simulink model "integration_PID_model_3"  (R2023a)
settings: Solver=VariableStepAuto  StartTime=0.0  StopTime=30  FixedStep=1e-3  RelTol=1e-3
PreLoadFcn:
  | %
  | 
  | %   Copyright 2020-2022 The MathWorks, Inc.
  | 
  | %Based on the quadcopter model used in jMAVSim
  | 
  | Ixx = 0.005; %Kgm^2
  | Iyy = 0.005;
  | Izz = 0.009;
  | 
  | 
  | inertia = diag([Ixx, Iyy, Izz]);
  | 
  | mass = 0.8; %Kg
  | g = 9.81; %m/s^2
  | 
  | armLength = 0.33/2; % length of Arm measured from center in m
  | 
  | rotorThrustMax = 4; %N
  | 
  | rotorTorqueMax = 0.05 ;%Nm
  | 
  | rotorTimeConst = 0.005 ;% time constant of rotor (motor + propeller)
  | 
  | %rotorOffset = [0 0 0]; % Rotors position offsets from Gravity center
  | 
  | dragCoeffMov = 0.01; %drag coefficient for linear motion of quadcopter
  | windVel = [0 0 0]';
  | 
  | % Initial states
  | init.posNED = [0, 0, 0]; % m
  | init.vb = [0 0 0]'; %m/s
  | init.euler = [0, 0, 0]'; %Roll Pitch Yaw Rads
  | init.angRates = [0, 0, 0]; %rad/s
  | 
  | 
  | %Computed from above values
  | rotorPositions = zeros(3,4);
  | axisD = armLength/sqrt(2);
  | rotorPositions(:,1) = [axisD, axisD, 0]';
  | rotorPositions(:,2) = [-axisD, -axisD, 0]';
  | rotorPositions(:,3) = [+axisD, -axisD, 0]';
  | rotorPositions(:,4) = [-axisD, axisD, 0]';
  | rotorDir = [-1, -1, 1, 1]; %rotation direction. +ve = clockwise
  | 
  | % Sample Time
  | SampleTime = 0.008;
  | 
  | %Gain to convert m to mm
  | m_to_mm = 1000;
  | 
  | %Gain to convert m/s^2 to mG
  | ms2_to_mg = (1/9.80665)*1000;
  | 
  | %Gain to convert m/s to cm/s
  | ms_to_cms = 100;
  | 
  | %Reference height for 'Flat Earth to LLA'
  | ref_height = -71.3232;
  | 
  | ... (+137 lines)
values from neighbouring files (symbols this model uses):
  delay_tilt = 0.004    [integration_parameters.m]    (also in simulation_parameters.m)
  kf = 65    [integration_parameters.m]    (also in simulation_parameters.m)
  Lh = 0.2    [CoG_shift.m]    (also in integration_parameters.m; simulation_parameters.m)
  Lv = 0.2    [integration_parameters.m]    (also in simulation_parameters.m)
  m = 1.12    [integration_parameters.m]    (also in optimal_controller_pitching.m; simulation_parameters.m)
  N = 150    [MPC_controller_full.m]
  p_D = 0    [controller_parameters.m]    (also in integration_parameters.m)
  p_I = 0    [controller_parameters.m]    (also in integration_parameters.m)
  p_P = 0.35    [controller_parameters.m]    (also in integration_parameters.m)
  pitch_D = 0    [controller_parameters.m]    (also in integration_parameters.m)
  pitch_I = 0.05    [controller_parameters.m]    (also in integration_parameters.m = 0)
  pitch_P = 2    [controller_parameters.m]    (also in integration_parameters.m = 10)
  q_D = 0    [controller_parameters.m]    (also in integration_parameters.m)
  q_I = 0    [controller_parameters.m]    (also in integration_parameters.m)
  q_P = 1.5    [controller_parameters.m]    (also in integration_parameters.m = 10)
  r_D = 0    [controller_parameters.m]    (also in integration_parameters.m)
  r_I = 0    [controller_parameters.m]    (also in integration_parameters.m)
  r_P = 1    [controller_parameters.m]    (also in integration_parameters.m)
  reference = [1 1 1 0 30 60]'    [integration_parameters.m]    (also in simulation_parameters.m = [1 1 1 0 30 40]')
  roll_D = 1    [controller_parameters.m]    (also in integration_parameters.m)
  roll_I = 0    [controller_parameters.m]    (also in integration_parameters.m)
  roll_P = 8    [controller_parameters.m]    (also in integration_parameters.m)
  s_r = [1 1 1 1 1 1]    [integration_parameters.m]    (also in simulation_parameters.m)
  Tmax = 5.5    [integration_parameters.m]    (also in simulation_parameters.m)
  vx_D = 0    [controller_parameters.m]
  vx_I = 0    [controller_parameters.m]
  vx_P = 10    [controller_parameters.m]
  vy_D = 0    [controller_parameters.m]    (also in integration_parameters.m)
  vy_I = 0    [controller_parameters.m]    (also in integration_parameters.m)
  vy_P = 12    [controller_parameters.m]    (also in integration_parameters.m)
  vz_D = 0    [controller_parameters.m]    (also in integration_parameters.m)
  vz_I = 0    [controller_parameters.m]    (also in integration_parameters.m)
  vz_P = 8    [controller_parameters.m]    (also in integration_parameters.m = 9)
  x_D = 1.5    [controller_parameters.m]    (also in integration_parameters.m = 0)
  x_I = 0    [controller_parameters.m]    (also in integration_parameters.m)
  x_P = 6    [controller_parameters.m]    (also in integration_parameters.m = 1.5)
  y_D = 0.3    [controller_parameters.m]    (also in integration_parameters.m)
  y_I = 0    [controller_parameters.m]    (also in integration_parameters.m)
  y_P = 1.5    [controller_parameters.m]    (also in integration_parameters.m)
  yaw_D = 0    [controller_parameters.m]    (also in integration_parameters.m)
  yaw_I = 0    [controller_parameters.m]    (also in integration_parameters.m)
  yaw_P = 1.5    [controller_parameters.m]    (also in integration_parameters.m)
  z_D = 0    [controller_parameters.m]    (also in integration_parameters.m)
  z_I = 0    [controller_parameters.m]    (also in integration_parameters.m)
  z_P = 3    [controller_parameters.m]    (also in integration_parameters.m = 2.5)
undefined symbols (not defined in the file or in its folder): X, Y, Z
libraries: sm_lib x47, nesl_utility x23, slpidlib x12, simulink x5, simulink_extras x4, SignalEditorBlockLib x1
(part 2 of 4)

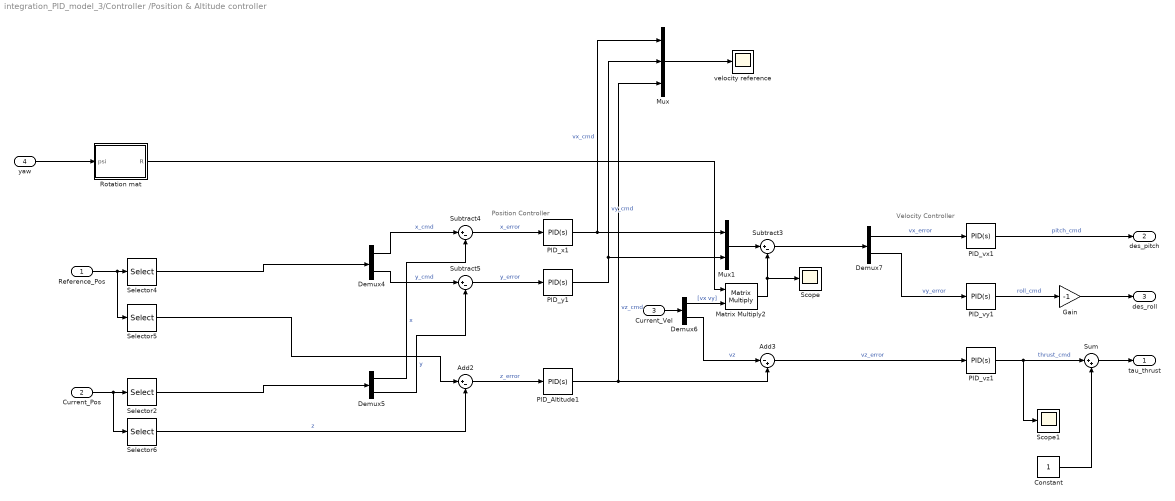
== system integration_PID_model_3/Controller /Position & Altitude controller ==
  note: Position Controller
  note: Velocity Controller
  Reference_Pos : Inport
  Current_Pos : Inport  Port=2
  Current_Vel : Inport  Port=3
  yaw : Inport  Port=4
  Add2 : Sum  Inputs=|+-
  Add3 : Sum  Inputs=|-+
  Constant : Constant
  Demux4 : Demux  Outputs=2
  Demux5 : Demux  Outputs=2
  Demux6 : Demux  Outputs=[2 1]
  Demux7 : Demux  Outputs=2
  Gain : Gain  Gain=-1
  Matrix Multiply2 : Product  Multiplication=Matrix(*)
  Mux : Mux  Inputs=3
  Mux1 : Mux  Inputs=2
  PID_Altitude1 : slpidlib/PID Controller  Controller=PID  Form=Parallel  TimeDomain=Continuous-time  UseExternalTs=off  SampleTime=-1  IntegratorMethod=Backward Euler  FilterMethod=Forward Euler  ControllerParametersSource=internal  P=z_P  I=z_I  UseKiTs=off  D=z_D  N=100  UseFilter=on  TunerSelectOption=Transfer Function Based (PID Tuner App)  InitialConditionSource=internal  InitialConditionForIntegrator=0  InitialConditionForFilter=0  DifferentiatorICPrevScaledInput=0  ExternalReset=none  TrackingMode=off  Kt=1  LimitOutput=on  SatLimitsSource=internal  UpperSaturationLimit=10  LowerSaturationLimit=-10  LinearizeAsGain=off  AntiWindupMode=clamping  Kb=1  LimitIntegrator=off  UpperIntegratorSaturationLimit=inf  LowerIntegratorSaturationLimit=-inf  POutMin=[]  POutMax=[]  IOutMin=[]  IOutMax=[]  DOutMin=[]  DOutMax=[]  NOutMin=[]  NOutMax=[]  SumOutMin=[]  SumOutMax=[]  SaturationOutMin=[]  SaturationOutMax=[]  PParamMin=[]  PParamMax=[]  IParamMin=[]  IParamMax=[]  DParamMin=[]  DParamMax=[]  NParamMin=[]  NParamMax=[]  KbParamMin=[]  KbParamMax=[]  KtParamMin=[]  KtParamMax=[]  KbOutMin=[]  KbOutMax=[]  KtOutMin=[]  KtOutMax=[]  IntegratorOutMin=[]  IntegratorOutMax=[]  FilterOutMin=[]  FilterOutMax=[]  SumI1OutMin=[]  SumI1OutMax=[]  SumI2OutMin=[]  SumI2OutMax=[]  SumI3OutMin=[]  SumI3OutMax=[]  SumI4OutMin=[]  SumI4OutMax=[]  SumDOutMin=[]  SumDOutMax=[]  DifferentiatorOutMin=[]  DifferentiatorOutMax=[]  FilterDiffOutCoefMin=[]  FilterDiffOutCoefMax=[]  ReciprocalOutMin=[]  ReciprocalOutMax=[]  SumDenOutMin=[]  SumDenOutMax=[]  SumNumOutMin=[]  SumNumOutMax=[]  DivideOutMin=[]  DivideOutMax=[]  UdiffTsProdOutMin=[]  UdiffTsProdOutMax=[]  NTsProdOutMin=[]  NTsProdOutMax=[]  UintegralTsProdOutMin=[]  UintegralTsProdOutMax=[]  UngainTsProdOutMin=[]  UngainTsProdOutMax=[]  ClampingZeroOutDataTypeStr=Inherit: Inherit via back propagation  ClampingZeroOutMin=[]  ClampingZeroOutMax=[]  FilterDenConstantOutDataTypeStr=Inherit: Inherit via back propagation  FilterDenConstantOutMin=[]  FilterDenConstantOutMax=[]  PCopyOutDataTypeStr=Inherit: Inherit via back propagation  PCopyOutMin=[]  PCopyOutMax=[]  NCopyOutDataTypeStr=Inherit: Inherit via back propagation  NCopyOutMin=[]  NCopyOutMax=[]  IntegratorContinuousStateAttributes=''  IntegratorStateMustResolveToSignalObject=off  IntegratorRTWStateStorageClass=Auto  FilterContinuousStateAttributes=''  FilterStateMustResolveToSignalObject=off  FilterRTWStateStorageClass=Auto  ParallelPVariant=InternalParameters  IdealPVariant=Disabled  IVariant=InternalParameters  DVariant=InternalParameters  IntegratorVariant=Continuous  SatVariant=Enabled  AWVariant=ContClampingParallel  PCopyVariant=Disabled  TRVariant=Disabled  FdbkBlocksVariant=Forward  IdealPFdbkVariant=Disabled  SatFdbkVariant=Disabled  DerivativeFilterVariant=ContFilter  NVariant=InternalParameters  NCopyVariant=Disabled  FilterICVariant=InternalICsFilter  IntegratorICVariant=InternalICs  ExternalResetVariant=Disabled  TRSumVariant=Passthrough  SumFdbkVariant=Disabled  SumVariant=Sum_PID  TsampFilterVariant=InternalTs  TsampNgainVariant=Passthrough  TsampIntegralVariant=Disabled_SignalSpec  ExternalSaturationOutDataTypeStr=Inherit: Same as second input
  PID_vx1 : slpidlib/PID Controller  Controller=PID  Form=Parallel  TimeDomain=Continuous-time  UseExternalTs=off  SampleTime=-1  IntegratorMethod=Forward Euler  FilterMethod=Forward Euler  ControllerParametersSource=internal  P=vx_P  I=vx_I  UseKiTs=off  D=vx_D  N=100  UseFilter=on  TunerSelectOption=Transfer Function Based (PID Tuner App)  InitialConditionSource=internal  InitialConditionForIntegrator=0  InitialConditionForFilter=0  DifferentiatorICPrevScaledInput=0  ExternalReset=none  TrackingMode=off  Kt=1  LimitOutput=on  SatLimitsSource=internal  UpperSaturationLimit=50  LowerSaturationLimit=-50  LinearizeAsGain=off  AntiWindupMode=none  Kb=1  LimitIntegrator=off  UpperIntegratorSaturationLimit=inf  LowerIntegratorSaturationLimit=-inf  POutMin=[]  POutMax=[]  IOutMin=[]  IOutMax=[]  DOutMin=[]  DOutMax=[]  NOutMin=[]  NOutMax=[]  SumOutMin=[]  SumOutMax=[]  SaturationOutMin=[]  SaturationOutMax=[]  PParamMin=[]  PParamMax=[]  IParamMin=[]  IParamMax=[]  DParamMin=[]  DParamMax=[]  NParamMin=[]  NParamMax=[]  KbParamMin=[]  KbParamMax=[]  KtParamMin=[]  KtParamMax=[]  KbOutMin=[]  KbOutMax=[]  KtOutMin=[]  KtOutMax=[]  IntegratorOutMin=[]  IntegratorOutMax=[]  FilterOutMin=[]  FilterOutMax=[]  SumI1OutMin=[]  SumI1OutMax=[]  SumI2OutMin=[]  SumI2OutMax=[]  SumI3OutMin=[]  SumI3OutMax=[]  SumI4OutMin=[]  SumI4OutMax=[]  SumDOutMin=[]  SumDOutMax=[]  DifferentiatorOutMin=[]  DifferentiatorOutMax=[]  FilterDiffOutCoefMin=[]  FilterDiffOutCoefMax=[]  ReciprocalOutMin=[]  ReciprocalOutMax=[]  SumDenOutMin=[]  SumDenOutMax=[]  SumNumOutMin=[]  SumNumOutMax=[]  DivideOutMin=[]  DivideOutMax=[]  UdiffTsProdOutMin=[]  UdiffTsProdOutMax=[]  NTsProdOutMin=[]  NTsProdOutMax=[]  UintegralTsProdOutMin=[]  UintegralTsProdOutMax=[]  UngainTsProdOutMin=[]  UngainTsProdOutMax=[]  ClampingZeroOutDataTypeStr=Inherit: Inherit via back propagation  ClampingZeroOutMin=[]  ClampingZeroOutMax=[]  FilterDenConstantOutDataTypeStr=Inherit: Inherit via back propagation  FilterDenConstantOutMin=[]  FilterDenConstantOutMax=[]  PCopyOutDataTypeStr=Inherit: Inherit via back propagation  PCopyOutMin=[]  PCopyOutMax=[]  NCopyOutDataTypeStr=Inherit: Inherit via back propagation  NCopyOutMin=[]  NCopyOutMax=[]  IntegratorContinuousStateAttributes=''  IntegratorStateMustResolveToSignalObject=off  IntegratorRTWStateStorageClass=Auto  FilterContinuousStateAttributes=''  FilterStateMustResolveToSignalObject=off  FilterRTWStateStorageClass=Auto  ParallelPVariant=InternalParameters  IdealPVariant=Disabled  IVariant=InternalParameters  DVariant=InternalParameters  IntegratorVariant=Continuous  SatVariant=Enabled  AWVariant=Passthrough  PCopyVariant=Disabled  TRVariant=Disabled  FdbkBlocksVariant=Forward  IdealPFdbkVariant=Disabled  SatFdbkVariant=Disabled  DerivativeFilterVariant=ContFilter  NVariant=InternalParameters  NCopyVariant=Disabled  FilterICVariant=InternalICsFilter  IntegratorICVariant=InternalICs  ExternalResetVariant=Disabled  TRSumVariant=Passthrough  SumFdbkVariant=Disabled  SumVariant=Sum_PID  TsampFilterVariant=InternalTs  TsampNgainVariant=Passthrough  TsampIntegralVariant=Disabled_SignalSpec  ExternalSaturationOutDataTypeStr=Inherit: Same as second input
  PID_vy1 : slpidlib/PID Controller  Controller=PID  Form=Parallel  TimeDomain=Continuous-time  UseExternalTs=off  SampleTime=-1  IntegratorMethod=Forward Euler  FilterMethod=Forward Euler  ControllerParametersSource=internal  P=vy_P  I=vy_I  UseKiTs=off  D=vy_D  N=100  UseFilter=on  TunerSelectOption=Frequency Response Based  InitialConditionSource=internal  InitialConditionForIntegrator=0  InitialConditionForFilter=0  DifferentiatorICPrevScaledInput=0  ExternalReset=none  TrackingMode=off  Kt=1  LimitOutput=on  SatLimitsSource=internal  UpperSaturationLimit=50  LowerSaturationLimit=-50  LinearizeAsGain=off  AntiWindupMode=none  Kb=1  LimitIntegrator=off  UpperIntegratorSaturationLimit=inf  LowerIntegratorSaturationLimit=-inf  POutMin=[]  POutMax=[]  IOutMin=[]  IOutMax=[]  DOutMin=[]  DOutMax=[]  NOutMin=[]  NOutMax=[]  SumOutMin=[]  SumOutMax=[]  SaturationOutMin=[]  SaturationOutMax=[]  PParamMin=[]  PParamMax=[]  IParamMin=[]  IParamMax=[]  DParamMin=[]  DParamMax=[]  NParamMin=[]  NParamMax=[]  KbParamMin=[]  KbParamMax=[]  KtParamMin=[]  KtParamMax=[]  KbOutMin=[]  KbOutMax=[]  KtOutMin=[]  KtOutMax=[]  IntegratorOutMin=[]  IntegratorOutMax=[]  FilterOutMin=[]  FilterOutMax=[]  SumI1OutMin=[]  SumI1OutMax=[]  SumI2OutMin=[]  SumI2OutMax=[]  SumI3OutMin=[]  SumI3OutMax=[]  SumI4OutMin=[]  SumI4OutMax=[]  SumDOutMin=[]  SumDOutMax=[]  DifferentiatorOutMin=[]  DifferentiatorOutMax=[]  FilterDiffOutCoefMin=[]  FilterDiffOutCoefMax=[]  ReciprocalOutMin=[]  ReciprocalOutMax=[]  SumDenOutMin=[]  SumDenOutMax=[]  SumNumOutMin=[]  SumNumOutMax=[]  DivideOutMin=[]  DivideOutMax=[]  UdiffTsProdOutMin=[]  UdiffTsProdOutMax=[]  NTsProdOutMin=[]  NTsProdOutMax=[]  UintegralTsProdOutMin=[]  UintegralTsProdOutMax=[]  UngainTsProdOutMin=[]  UngainTsProdOutMax=[]  ClampingZeroOutDataTypeStr=Inherit: Inherit via back propagation  ClampingZeroOutMin=[]  ClampingZeroOutMax=[]  FilterDenConstantOutDataTypeStr=Inherit: Inherit via back propagation  FilterDenConstantOutMin=[]  FilterDenConstantOutMax=[]  PCopyOutDataTypeStr=Inherit: Inherit via back propagation  PCopyOutMin=[]  PCopyOutMax=[]  NCopyOutDataTypeStr=Inherit: Inherit via back propagation  NCopyOutMin=[]  NCopyOutMax=[]  IntegratorContinuousStateAttributes=''  IntegratorStateMustResolveToSignalObject=off  IntegratorRTWStateStorageClass=Auto  FilterContinuousStateAttributes=''  FilterStateMustResolveToSignalObject=off  FilterRTWStateStorageClass=Auto  ParallelPVariant=InternalParameters  IdealPVariant=Disabled  IVariant=InternalParameters  DVariant=InternalParameters  IntegratorVariant=Continuous  SatVariant=Enabled  AWVariant=Passthrough  PCopyVariant=Disabled  TRVariant=Disabled  FdbkBlocksVariant=Forward  IdealPFdbkVariant=Disabled  SatFdbkVariant=Disabled  DerivativeFilterVariant=ContFilter  NVariant=InternalParameters  NCopyVariant=Disabled  FilterICVariant=InternalICsFilter  IntegratorICVariant=InternalICs  ExternalResetVariant=Disabled  TRSumVariant=Passthrough  SumFdbkVariant=Disabled  SumVariant=Sum_PID  TsampFilterVariant=InternalTs  TsampNgainVariant=Passthrough  TsampIntegralVariant=Disabled_SignalSpec  ExternalSaturationOutDataTypeStr=Inherit: Same as second input
  PID_vz1 : slpidlib/PID Controller  Controller=PID  Form=Parallel  TimeDomain=Continuous-time  UseExternalTs=off  SampleTime=-1  IntegratorMethod=Backward Euler  FilterMethod=Forward Euler  ControllerParametersSource=internal  P=vz_P  I=vz_I  UseKiTs=off  D=vz_D  N=100  UseFilter=on  TunerSelectOption=Transfer Function Based (PID Tuner App)  InitialConditionSource=internal  InitialConditionForIntegrator=0  InitialConditionForFilter=0  DifferentiatorICPrevScaledInput=0  ExternalReset=none  TrackingMode=off  Kt=1  LimitOutput=off  SatLimitsSource=internal  UpperSaturationLimit=2  LowerSaturationLimit=0  LinearizeAsGain=off  AntiWindupMode=none  Kb=1  LimitIntegrator=off  UpperIntegratorSaturationLimit=inf  LowerIntegratorSaturationLimit=-inf  POutMin=[]  POutMax=[]  IOutMin=[]  IOutMax=[]  DOutMin=[]  DOutMax=[]  NOutMin=[]  NOutMax=[]  SumOutMin=[]  SumOutMax=[]  SaturationOutMin=[]  SaturationOutMax=[]  PParamMin=[]  PParamMax=[]  IParamMin=[]  IParamMax=[]  DParamMin=[]  DParamMax=[]  NParamMin=[]  NParamMax=[]  KbParamMin=[]  KbParamMax=[]  KtParamMin=[]  KtParamMax=[]  KbOutMin=[]  KbOutMax=[]  KtOutMin=[]  KtOutMax=[]  IntegratorOutMin=[]  IntegratorOutMax=[]  FilterOutMin=[]  FilterOutMax=[]  SumI1OutMin=[]  SumI1OutMax=[]  SumI2OutMin=[]  SumI2OutMax=[]  SumI3OutMin=[]  SumI3OutMax=[]  SumI4OutMin=[]  SumI4OutMax=[]  SumDOutMin=[]  SumDOutMax=[]  DifferentiatorOutMin=[]  DifferentiatorOutMax=[]  FilterDiffOutCoefMin=[]  FilterDiffOutCoefMax=[]  ReciprocalOutMin=[]  ReciprocalOutMax=[]  SumDenOutMin=[]  SumDenOutMax=[]  SumNumOutMin=[]  SumNumOutMax=[]  DivideOutMin=[]  DivideOutMax=[]  UdiffTsProdOutMin=[]  UdiffTsProdOutMax=[]  NTsProdOutMin=[]  NTsProdOutMax=[]  UintegralTsProdOutMin=[]  UintegralTsProdOutMax=[]  UngainTsProdOutMin=[]  UngainTsProdOutMax=[]  ClampingZeroOutDataTypeStr=Inherit: Inherit via back propagation  ClampingZeroOutMin=[]  ClampingZeroOutMax=[]  FilterDenConstantOutDataTypeStr=Inherit: Inherit via back propagation  FilterDenConstantOutMin=[]  FilterDenConstantOutMax=[]  PCopyOutDataTypeStr=Inherit: Inherit via back propagation  PCopyOutMin=[]  PCopyOutMax=[]  NCopyOutDataTypeStr=Inherit: Inherit via back propagation  NCopyOutMin=[]  NCopyOutMax=[]  IntegratorContinuousStateAttributes=''  IntegratorStateMustResolveToSignalObject=off  IntegratorRTWStateStorageClass=Auto  FilterContinuousStateAttributes=''  FilterStateMustResolveToSignalObject=off  FilterRTWStateStorageClass=Auto  ParallelPVariant=InternalParameters  IdealPVariant=Disabled  IVariant=InternalParameters  DVariant=InternalParameters  IntegratorVariant=Continuous  SatVariant=Disabled  AWVariant=Passthrough  PCopyVariant=Disabled  TRVariant=Disabled  FdbkBlocksVariant=Forward  IdealPFdbkVariant=Disabled  SatFdbkVariant=Disabled  DerivativeFilterVariant=ContFilter  NVariant=InternalParameters  NCopyVariant=Disabled  FilterICVariant=InternalICsFilter  IntegratorICVariant=InternalICs  ExternalResetVariant=Disabled  TRSumVariant=Passthrough  SumFdbkVariant=Disabled  SumVariant=Sum_PID  TsampFilterVariant=InternalTs  TsampNgainVariant=Passthrough  TsampIntegralVariant=Disabled_SignalSpec  ExternalSaturationOutDataTypeStr=Inherit: Same as second input
  PID_x1 : slpidlib/PID Controller  Controller=PID  Form=Parallel  TimeDomain=Continuous-time  UseExternalTs=off  SampleTime=-1  IntegratorMethod=Forward Euler  FilterMethod=Forward Euler  ControllerParametersSource=internal  P=x_P  I=x_I  UseKiTs=off  D=x_D  N=100  UseFilter=on  TunerSelectOption=Frequency Response Based  InitialConditionSource=internal  InitialConditionForIntegrator=0  InitialConditionForFilter=0  DifferentiatorICPrevScaledInput=0  ExternalReset=none  TrackingMode=off  Kt=1  LimitOutput=on  SatLimitsSource=internal  UpperSaturationLimit=20  LowerSaturationLimit=-20  LinearizeAsGain=off  AntiWindupMode=clamping  Kb=1  LimitIntegrator=off  UpperIntegratorSaturationLimit=inf  LowerIntegratorSaturationLimit=-inf  POutMin=[]  POutMax=[]  IOutMin=[]  IOutMax=[]  DOutMin=[]  DOutMax=[]  NOutMin=[]  NOutMax=[]  SumOutMin=[]  SumOutMax=[]  SaturationOutMin=[]  SaturationOutMax=[]  PParamMin=[]  PParamMax=[]  IParamMin=[]  IParamMax=[]  DParamMin=[]  DParamMax=[]  NParamMin=[]  NParamMax=[]  KbParamMin=[]  KbParamMax=[]  KtParamMin=[]  KtParamMax=[]  KbOutMin=[]  KbOutMax=[]  KtOutMin=[]  KtOutMax=[]  IntegratorOutMin=[]  IntegratorOutMax=[]  FilterOutMin=[]  FilterOutMax=[]  SumI1OutMin=[]  SumI1OutMax=[]  SumI2OutMin=[]  SumI2OutMax=[]  SumI3OutMin=[]  SumI3OutMax=[]  SumI4OutMin=[]  SumI4OutMax=[]  SumDOutMin=[]  SumDOutMax=[]  DifferentiatorOutMin=[]  DifferentiatorOutMax=[]  FilterDiffOutCoefMin=[]  FilterDiffOutCoefMax=[]  ReciprocalOutMin=[]  ReciprocalOutMax=[]  SumDenOutMin=[]  SumDenOutMax=[]  SumNumOutMin=[]  SumNumOutMax=[]  DivideOutMin=[]  DivideOutMax=[]  UdiffTsProdOutMin=[]  UdiffTsProdOutMax=[]  NTsProdOutMin=[]  NTsProdOutMax=[]  UintegralTsProdOutMin=[]  UintegralTsProdOutMax=[]  UngainTsProdOutMin=[]  UngainTsProdOutMax=[]  ClampingZeroOutDataTypeStr=Inherit: Inherit via back propagation  ClampingZeroOutMin=[]  ClampingZeroOutMax=[]  FilterDenConstantOutDataTypeStr=Inherit: Inherit via back propagation  FilterDenConstantOutMin=[]  FilterDenConstantOutMax=[]  PCopyOutDataTypeStr=Inherit: Inherit via back propagation  PCopyOutMin=[]  PCopyOutMax=[]  NCopyOutDataTypeStr=Inherit: Inherit via back propagation  NCopyOutMin=[]  NCopyOutMax=[]  IntegratorContinuousStateAttributes=''  IntegratorStateMustResolveToSignalObject=off  IntegratorRTWStateStorageClass=Auto  FilterContinuousStateAttributes=''  FilterStateMustResolveToSignalObject=off  FilterRTWStateStorageClass=Auto  ParallelPVariant=InternalParameters  IdealPVariant=Disabled  IVariant=InternalParameters  DVariant=InternalParameters  IntegratorVariant=Continuous  SatVariant=Enabled  AWVariant=ContClampingParallel  PCopyVariant=Disabled  TRVariant=Disabled  FdbkBlocksVariant=Forward  IdealPFdbkVariant=Disabled  SatFdbkVariant=Disabled  DerivativeFilterVariant=ContFilter  NVariant=InternalParameters  NCopyVariant=Disabled  FilterICVariant=InternalICsFilter  IntegratorICVariant=InternalICs  ExternalResetVariant=Disabled  TRSumVariant=Passthrough  SumFdbkVariant=Disabled  SumVariant=Sum_PID  TsampFilterVariant=InternalTs  TsampNgainVariant=Passthrough  TsampIntegralVariant=Disabled_SignalSpec  ExternalSaturationOutDataTypeStr=Inherit: Same as second input
  PID_y1 : slpidlib/PID Controller  Controller=PID  Form=Parallel  TimeDomain=Continuous-time  UseExternalTs=off  SampleTime=-1  IntegratorMethod=Forward Euler  FilterMethod=Forward Euler  ControllerParametersSource=internal  P=y_P  I=y_I  UseKiTs=off  D=y_D  N=100  UseFilter=on  TunerSelectOption=Transfer Function Based (PID Tuner App)  InitialConditionSource=internal  InitialConditionForIntegrator=0  InitialConditionForFilter=0  DifferentiatorICPrevScaledInput=0  ExternalReset=none  TrackingMode=off  Kt=1  LimitOutput=on  SatLimitsSource=internal  UpperSaturationLimit=20  LowerSaturationLimit=-20  LinearizeAsGain=off  AntiWindupMode=clamping  Kb=1  LimitIntegrator=off  UpperIntegratorSaturationLimit=inf  LowerIntegratorSaturationLimit=-inf  POutMin=[]  POutMax=[]  IOutMin=[]  IOutMax=[]  DOutMin=[]  DOutMax=[]  NOutMin=[]  NOutMax=[]  SumOutMin=[]  SumOutMax=[]  SaturationOutMin=[]  SaturationOutMax=[]  PParamMin=[]  PParamMax=[]  IParamMin=[]  IParamMax=[]  DParamMin=[]  DParamMax=[]  NParamMin=[]  NParamMax=[]  KbParamMin=[]  KbParamMax=[]  KtParamMin=[]  KtParamMax=[]  KbOutMin=[]  KbOutMax=[]  KtOutMin=[]  KtOutMax=[]  IntegratorOutMin=[]  IntegratorOutMax=[]  FilterOutMin=[]  FilterOutMax=[]  SumI1OutMin=[]  SumI1OutMax=[]  SumI2OutMin=[]  SumI2OutMax=[]  SumI3OutMin=[]  SumI3OutMax=[]  SumI4OutMin=[]  SumI4OutMax=[]  SumDOutMin=[]  SumDOutMax=[]  DifferentiatorOutMin=[]  DifferentiatorOutMax=[]  FilterDiffOutCoefMin=[]  FilterDiffOutCoefMax=[]  ReciprocalOutMin=[]  ReciprocalOutMax=[]  SumDenOutMin=[]  SumDenOutMax=[]  SumNumOutMin=[]  SumNumOutMax=[]  DivideOutMin=[]  DivideOutMax=[]  UdiffTsProdOutMin=[]  UdiffTsProdOutMax=[]  NTsProdOutMin=[]  NTsProdOutMax=[]  UintegralTsProdOutMin=[]  UintegralTsProdOutMax=[]  UngainTsProdOutMin=[]  UngainTsProdOutMax=[]  ClampingZeroOutDataTypeStr=Inherit: Inherit via back propagation  ClampingZeroOutMin=[]  ClampingZeroOutMax=[]  FilterDenConstantOutDataTypeStr=Inherit: Inherit via back propagation  FilterDenConstantOutMin=[]  FilterDenConstantOutMax=[]  PCopyOutDataTypeStr=Inherit: Inherit via back propagation  PCopyOutMin=[]  PCopyOutMax=[]  NCopyOutDataTypeStr=Inherit: Inherit via back propagation  NCopyOutMin=[]  NCopyOutMax=[]  IntegratorContinuousStateAttributes=''  IntegratorStateMustResolveToSignalObject=off  IntegratorRTWStateStorageClass=Auto  FilterContinuousStateAttributes=''  FilterStateMustResolveToSignalObject=off  FilterRTWStateStorageClass=Auto  ParallelPVariant=InternalParameters  IdealPVariant=Disabled  IVariant=InternalParameters  DVariant=InternalParameters  IntegratorVariant=Continuous  SatVariant=Enabled  AWVariant=ContClampingParallel  PCopyVariant=Disabled  TRVariant=Disabled  FdbkBlocksVariant=Forward  IdealPFdbkVariant=Disabled  SatFdbkVariant=Disabled  DerivativeFilterVariant=ContFilter  NVariant=InternalParameters  NCopyVariant=Disabled  FilterICVariant=InternalICsFilter  IntegratorICVariant=InternalICs  ExternalResetVariant=Disabled  TRSumVariant=Passthrough  SumFdbkVariant=Disabled  SumVariant=Sum_PID  TsampFilterVariant=InternalTs  TsampNgainVariant=Passthrough  TsampIntegralVariant=Disabled_SignalSpec  ExternalSaturationOutDataTypeStr=Inherit: Same as second input
  "Rotation mat " : MATLAB Function  TreatAsAtomicUnit=on
  Scope : Scope
  Scope1 : Scope
  Selector2 : Selector  InputPortWidth=3  IndexOptions=Index vector (dialog)  Indices=[1 2]  OutputSizes=1
  Selector4 : Selector  InputPortWidth=3  IndexOptions=Index vector (dialog)  Indices=[1 2]  OutputSizes=1
  Selector5 : Selector  InputPortWidth=3  IndexOptions=Index vector (dialog)  Indices=[3]  OutputSizes=1
  Selector6 : Selector  InputPortWidth=3  IndexOptions=Index vector (dialog)  Indices=[3]  OutputSizes=1
  Subtract3 : Sum  Inputs=|+-
  Subtract4 : Sum  Inputs=|+-
  Subtract5 : Sum  Inputs=|+-
  Sum : Sum  Inputs=|++
  velocity reference : Scope
  tau_thrust : Outport
  des_pitch : Outport  Port=2
  des_roll : Outport  Port=3
  wires:
  Demux7/2 -> PID_vy1/1  "vy_error"
  Demux5/1 -> Subtract4/2  "x"
  PID_vy1/1 -> Gain/1  "roll_cmd"
  Demux5/2 -> Subtract5/2  "y"
  Demux6/2 -> Add3/1  "vz"
  Selector4/1 -> Demux4/1
  Subtract5/1 -> PID_y1/1  "y_error"
  Current_Vel/1 -> Demux6/1
  Demux7/1 -> PID_vx1/1  "vx_error"
  Mux1/1 -> Subtract3/1
  "Rotation mat "/1(R) -> Matrix Multiply2/1
  Add2/1 -> PID_Altitude1/1  "z_error"
  Demux4/2 -> Subtract5/1  "y_cmd"
  Subtract4/1 -> PID_x1/1  "x_error"
  Demux4/1 -> Subtract4/1  "x_cmd"
  PID_vx1/1 -> des_pitch/1  "pitch_cmd"
  PID_vz1/1 -> Sum/1, Scope1/1  "thrust_cmd"
  Selector2/1 -> Demux5/1
  Subtract3/1 -> Demux7/1
  Reference_Pos/1 -> Selector5/1, Selector4/1
  Selector5/1 -> Add2/1
  Current_Pos/1 -> Selector2/1, Selector6/1
  Selector6/1 -> Add2/2  "z"
  Demux6/1 -> Matrix Multiply2/2  "[vx vy]"
  Matrix Multiply2/1 -> Subtract3/2, Scope/1
  Add3/1 -> PID_vz1/1  "vz_error"
  PID_y1/1 -> Mux1/2, Mux/2  "vy_cmd"
  PID_x1/1 -> Mux1/1, Mux/1  "vx_cmd"
  PID_Altitude1/1 -> Add3/2, Mux/3  "vz_cmd"
  Mux/1 -> velocity reference/1
  Gain/1 -> des_roll/1
  yaw/1 -> "Rotation mat "/1(psi)
  Sum/1 -> tau_thrust/1
  Constant/1 -> Sum/2

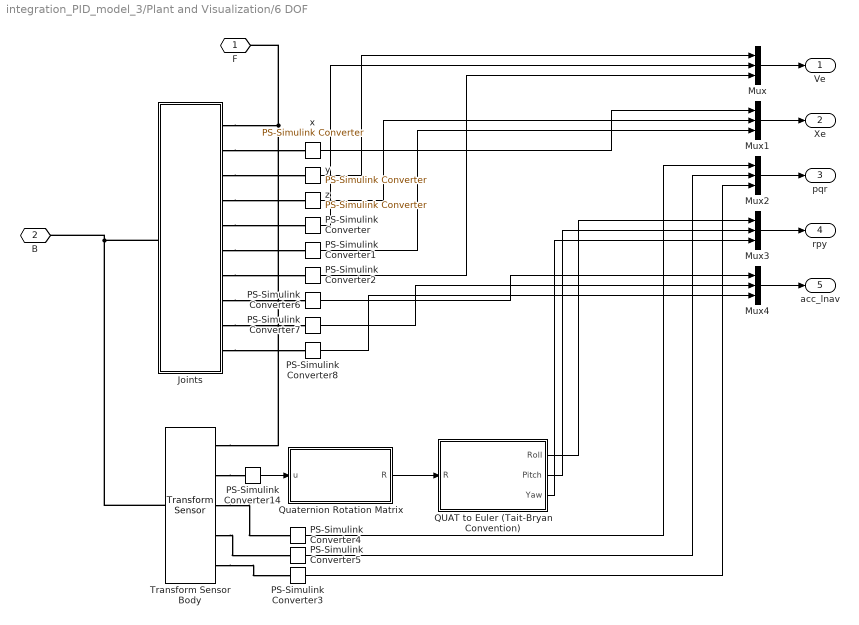
== system integration_PID_model_3/Plant and Visualization/6 DOF ==
  " QUAT to Euler (Tait-Bryan Convention)" : MATLAB Function  TreatAsAtomicUnit=on
  Joints : Subsystem
  Mux{,1..4} (5 alike) : Mux  Inputs=3
  PS-Simulink Converter{,1..2,4..5,14} (6 alike) : nesl_utility/PS-Simulink Converter  PhysicalDomain=network_engine_domain  SubClassName=ps_output  LeftPortType=input  RightPortType=output  PseudoPeriodic=off  Frequencies=[]  VectorFormat=1-D array  Unit=inherit  AffineConversion=off
  PS-Simulink Converter{3,6..8} (4 alike) : nesl_utility/PS-Simulink Converter  PhysicalDomain=network_engine_domain  SubClassName=ps_output  LeftPortType=input  RightPortType=output  PseudoPeriodic=off  Frequencies=[]  VectorFormat=1-D array  Unit=1  AffineConversion=off
  Quaternion Rotation Matrix : MATLAB Function  TreatAsAtomicUnit=on
  Transform Sensor Body : sm_lib/Frames and Transforms/Transform Sensor  MeasurementFrame=Follower  RotationSequence=XYX  SenseAngle=off  SenseAxis=off  SenseQ=on  SenseR=off  SenseRotationSequence=off  SenseOmegaX=on  SenseOmegaY=on  SenseOmegaZ=on  SenseQDot=off  SenseRDot=off  SenseRotationSequenceDot=off  SenseAlphaX=off  SenseAlphaY=off  SenseAlphaZ=off  SenseQDDot=off  SenseRDDot=off  SenseX=off  SenseY=off  SenseZ=off  SenseRad=off  SenseAzim=off  SenseDist=off  SenseInc=off  SenseXDot=off  SenseYDot=off  SenseZDot=off  SenseRadDot=off  SenseAzimDot=off  SenseDistDot=off  SenseIncDot=off  SenseXDDot=off  SenseYDDot=off  SenseZDDot=off  SenseRadDDot=off  SenseAzimDDot=off  SenseDistDDot=off  SenseIncDDot=off
  x : nesl_utility/PS-Simulink Converter  PhysicalDomain=network_engine_domain  SubClassName=ps_output  LeftPortType=input  RightPortType=output  PseudoPeriodic=off  Frequencies=[]  VectorFormat=1-D array  Unit=1  AffineConversion=off
  y : nesl_utility/PS-Simulink Converter  PhysicalDomain=network_engine_domain  SubClassName=ps_output  LeftPortType=input  RightPortType=output  PseudoPeriodic=off  Frequencies=[]  VectorFormat=1-D array  Unit=1  AffineConversion=off
  z : nesl_utility/PS-Simulink Converter  PhysicalDomain=network_engine_domain  SubClassName=ps_output  LeftPortType=input  RightPortType=output  PseudoPeriodic=off  Frequencies=[]  VectorFormat=1-D array  Unit=1  AffineConversion=off
  F : PMIOPort  Side=Left
  B : PMIOPort  Port=2  Side=Left
  Ve : Outport
  Xe : Outport  Port=2
  pqr : Outport  Port=3
  rpy : Outport  Port=4
  acc_lnav : Outport  Port=5
  wires:
  x/1 -> Mux1/1
  y/1 -> Mux/1
  PS-Simulink Converter3/1 -> Mux2/3
  PS-Simulink Converter6/1 -> Mux4/1
  Mux/1 -> Ve/1
  Mux1/1 -> Xe/1
  Mux3/1 -> rpy/1
  Mux4/1 -> acc_lnav/1
  PS-Simulink Converter/1 -> Mux/2
  z/1 -> Mux1/2
  PS-Simulink Converter4/1 -> Mux2/1
  PS-Simulink Converter7/1 -> Mux4/2
  PS-Simulink Converter8/1 -> Mux4/3
  PS-Simulink Converter2/1 -> Mux/3
  PS-Simulink Converter1/1 -> Mux1/3
  PS-Simulink Converter5/1 -> Mux2/2
  Quaternion Rotation Matrix/1(R) -> " QUAT to Euler (Tait-Bryan Convention)"/1(R)
  PS-Simulink Converter14/1 -> Quaternion Rotation Matrix/1(u)
  " QUAT to Euler (Tait-Bryan Convention)"/1(Roll) -> Mux3/1
  " QUAT to Euler (Tait-Bryan Convention)"/2(Pitch) -> Mux3/2
  " QUAT to Euler (Tait-Bryan Convention)"/3(Yaw) -> Mux3/3
  Mux2/1 -> pqr/1
  connections:
  Transform Sensor Body/RConn1 -- Joints/RConn1 -- F/RConn1
  Joints/RConn2 -- x/LConn1
  Joints/RConn3 -- y/LConn1
  Transform Sensor Body/LConn1 -- B/RConn1 -- Joints/LConn1
  Joints/RConn4 -- z/LConn1
  Joints/RConn5 -- PS-Simulink Converter/LConn1
  Joints/RConn6 -- PS-Simulink Converter1/LConn1
  Joints/RConn7 -- PS-Simulink Converter2/LConn1
  Joints/RConn8 -- PS-Simulink Converter6/LConn1
  Joints/RConn9 -- PS-Simulink Converter7/LConn1
  Joints/RConn10 -- PS-Simulink Converter8/LConn1
  Transform Sensor Body/RConn2 -- PS-Simulink Converter14/LConn1
  Transform Sensor Body/RConn3 -- PS-Simulink Converter4/LConn1
  Transform Sensor Body/RConn4 -- PS-Simulink Converter5/LConn1
  Transform Sensor Body/RConn5 -- PS-Simulink Converter3/LConn1
